simulink model "stability_controller_testbench"  (R2022b)
settings: Solver=VariableStepAuto  StartTime=0.0  StopTime=sim_t_stop  RelTol=1e-3
undefined symbols (not defined in the file): A, B, beta_off_deg, beta_on_deg, C, D, delta_base_deg, delta_base_t_on, delta_extra_deg, delta_extra_t_off, delta_extra_t_on, G_rref, Ki_beta, Ki_r, Kp_beta, Kp_r, Mz_max, Mz_min, psi0, Vx_scenario, X0, x0_lat, Y0
libraries: slpidlib x2
settings Model: Creator=joseg  LastModifiedBy=joseg
settings OptimizationCC: ReuseModelBlockBuffer=on

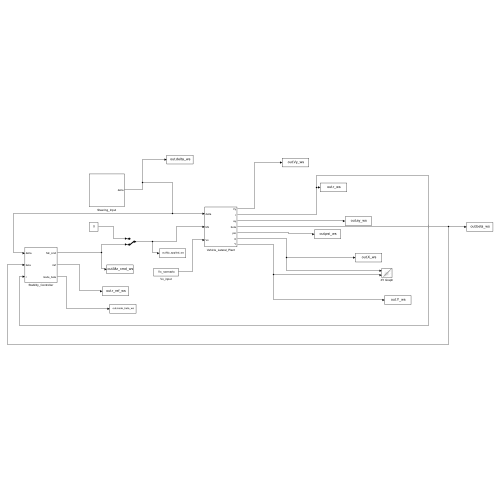
[thumbnail: Simulink's stored preview of the top-level diagram]
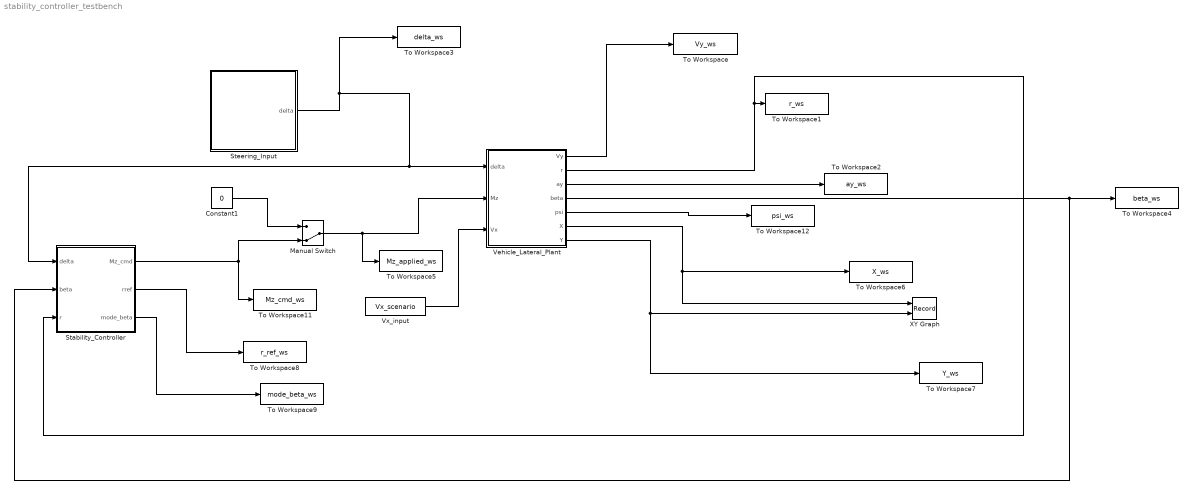
== system stability_controller_testbench ==
  Constant1 : Constant  Value=0
  Manual Switch : ManualSwitch  CurrentSetting=0
  Stability_Controller : Subsystem
  Steering_Input : Subsystem
  To Workspace : ToWorkspace  VariableName=Vy_ws  SaveFormat=Structure With Time  SampleTime=-1
      settings: Save2DSignal=2-D array (concatenate along first dimension)
  To Workspace1 : ToWorkspace  VariableName=r_ws  SaveFormat=Structure With Time  SampleTime=-1
      settings: Save2DSignal=2-D array (concatenate along first dimension)
  To Workspace11 : ToWorkspace  VariableName=Mz_cmd_ws  SaveFormat=Structure With Time  SampleTime=-1
      settings: Save2DSignal=2-D array (concatenate along first dimension)
  To Workspace12 : ToWorkspace  VariableName=psi_ws  SaveFormat=Structure With Time  SampleTime=-1
      settings: Save2DSignal=2-D array (concatenate along first dimension)
  To Workspace2 : ToWorkspace  VariableName=ay_ws  SaveFormat=Structure With Time  SampleTime=-1
      settings: Save2DSignal=2-D array (concatenate along first dimension)
  To Workspace3 : ToWorkspace  VariableName=delta_ws  SaveFormat=Structure With Time  SampleTime=-1
      settings: Save2DSignal=2-D array (concatenate along first dimension)
  To Workspace4 : ToWorkspace  VariableName=beta_ws  SaveFormat=Structure With Time  SampleTime=-1
      settings: Save2DSignal=2-D array (concatenate along first dimension)
  To Workspace5 : ToWorkspace  VariableName=Mz_applied_ws  SaveFormat=Structure With Time  SampleTime=-1
      settings: Save2DSignal=2-D array (concatenate along first dimension)
  To Workspace6 : ToWorkspace  VariableName=X_ws  SaveFormat=Structure With Time  SampleTime=-1
      settings: Save2DSignal=2-D array (concatenate along first dimension)
  To Workspace7 : ToWorkspace  VariableName=Y_ws  SaveFormat=Structure With Time  SampleTime=-1
      settings: Save2DSignal=2-D array (concatenate along first dimension)
  To Workspace8 : ToWorkspace  VariableName=r_ref_ws  SaveFormat=Structure With Time  SampleTime=-1
      settings: Save2DSignal=2-D array (concatenate along first dimension)
  To Workspace9 : ToWorkspace  VariableName=mode_beta_ws  SaveFormat=Structure With Time  SampleTime=-1
      settings: Save2DSignal=2-D array (concatenate along first dimension)
  Vehicle_Lateral_Plant : Subsystem
  Vx_input : Constant  Value=Vx_scenario
  XY Graph : Record  FileSettingsInternal="{\"entries\":[{\"content\":{\"excelSettings\":{\"content\":{},\"type\":\"Streamout.ExcelSettings\"}},\"type\":\"Streamout.FileSettingStorage\",\"uuid\":\"\"}],\"packageUris\":[\"http:\\/\\/schema.mathworks.com\\/mf0\\/streamout_blocks\\/R2020a\"],\"version\":\"1.0\"}"  Layout=[1 1]  SignalsInternal="{\"entries\":[{\"content\":{\"signals\":[{\"content\":{\"blockPath\":[],\"dimensions\":[1],\"domain\":\"\",\"lineColor\":\"#77ac30\",\"port\":1,\"signalID\":1,\"signalName\":\"Vehicle_Lateral_Plant:6\"},\"type\":\"RecordBlkView.Signal\",\"uuid\":\"\"},{\"content\":{\"blockPath\":[],\"dimensions\":[1],\"domain\":\"\",\"lineColor\":\"#4dbeee\",\"port\":2,\"signalID\":2,\"signalName\":\"Vehicle_Lateral_Plant:7\"},\"type\":\"RecordBlkView.Signal\",\"uuid\":\"\"}]},\"type\":\"RecordBlkView.InputSignals\",\"uuid\":\"\"}],\"packageUris\":[\"http:\\/\\/schema.mathworks.com\\/mf0\\/streamout_blocks\\/R2020a\"],\"version\":\"1.0\"}"  VisualizationBindings="{\"xyplotplugin\":{\"info\":[{\"series\":[],\"subplotID\":1}]}}"  CompatibilityTag=XY
  wires:
  Steering_Input/1(delta) -> To Workspace3/1, Stability_Controller/1(delta), Vehicle_Lateral_Plant/1(delta)
  Vehicle_Lateral_Plant/4(beta) -> Stability_Controller/2(beta), To Workspace4/1
  Vehicle_Lateral_Plant/7(Y) -> XY Graph/2, To Workspace7/1
  Vehicle_Lateral_Plant/1(Vy) -> To Workspace/1
  Vehicle_Lateral_Plant/6(X) -> XY Graph/1, To Workspace6/1
  Vehicle_Lateral_Plant/3(ay) -> To Workspace2/1
  Vx_input/1 -> Vehicle_Lateral_Plant/3(Vx)
  Vehicle_Lateral_Plant/5(psi) -> To Workspace12/1
  Stability_Controller/1(Mz_cmd) -> Manual Switch/2, To Workspace11/1
  Stability_Controller/2(rref) -> To Workspace8/1
  Stability_Controller/3(mode_beta) -> To Workspace9/1
  Vehicle_Lateral_Plant/2(r) -> Stability_Controller/3(r), To Workspace1/1
  Constant1/1 -> Manual Switch/1
  Manual Switch/1 -> To Workspace5/1, Vehicle_Lateral_Plant/2(Mz)

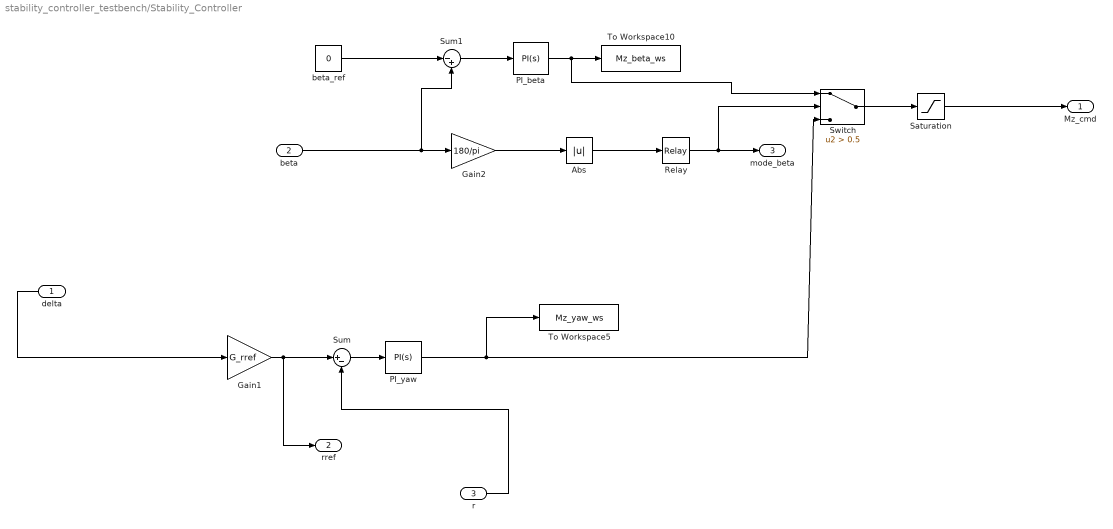
== system stability_controller_testbench/Stability_Controller ==
  delta : Inport
  beta : Inport  Port=2
  r : Inport  Port=3
  Abs : Abs  SaturateOnIntegerOverflow=off
  Gain1 : Gain  Gain=G_rref
  Gain2 : Gain  Gain=180/pi
  PI_beta : slpidlib/PID Controller  Controller=PI  Form=Parallel  TimeDomain=Continuous-time  UseExternalTs=off  SampleTime=-1  IntegratorMethod=Forward Euler  FilterMethod=Forward Euler  ControllerParametersSource=internal  P=Kp_beta  I=Ki_beta  UseKiTs=off  D=0  N=100  UseFilter=on  TunerSelectOption=Transfer Function Based (PID Tuner App)  InitialConditionSource=internal  InitialConditionForIntegrator=0  InitialConditionForFilter=0  DifferentiatorICPrevScaledInput=0  ExternalReset=none  TrackingMode=off  Kt=1  LimitOutput=off  SatLimitsSource=internal  UpperSaturationLimit=inf  LowerSaturationLimit=-inf  LinearizeAsGain=on  AntiWindupMode=none  Kb=1  LimitIntegrator=off  UpperIntegratorSaturationLimit=inf  LowerIntegratorSaturationLimit=-inf  POutMin=[]  POutMax=[]  IOutMin=[]  IOutMax=[]  DOutMin=[]  DOutMax=[]  NOutMin=[]  NOutMax=[]  SumOutMin=[]  SumOutMax=[]  SaturationOutMin=[]  SaturationOutMax=[]  PParamMin=[]  PParamMax=[]  IParamMin=[]  IParamMax=[]  DParamMin=[]  DParamMax=[]  NParamMin=[]  NParamMax=[]  KbParamMin=[]  KbParamMax=[]  KtParamMin=[]  KtParamMax=[]  KbOutMin=[]  KbOutMax=[]  KtOutMin=[]  KtOutMax=[]  IntegratorOutMin=[]  IntegratorOutMax=[]  FilterOutMin=[]  FilterOutMax=[]  SumI1OutMin=[]  SumI1OutMax=[]  SumI2OutMin=[]  SumI2OutMax=[]  SumI3OutMin=[]  SumI3OutMax=[]  SumI4OutMin=[]  SumI4OutMax=[]  SumDOutMin=[]  SumDOutMax=[]  DifferentiatorOutMin=[]  DifferentiatorOutMax=[]  FilterDiffOutCoefMin=[]  FilterDiffOutCoefMax=[]  ReciprocalOutMin=[]  ReciprocalOutMax=[]  SumDenOutMin=[]  SumDenOutMax=[]  SumNumOutMin=[]  SumNumOutMax=[]  DivideOutMin=[]  DivideOutMax=[]  UdiffTsProdOutMin=[]  UdiffTsProdOutMax=[]  NTsProdOutMin=[]  NTsProdOutMax=[]  UintegralTsProdOutMin=[]  UintegralTsProdOutMax=[]  UngainTsProdOutMin=[]  UngainTsProdOutMax=[]  IntegratorContinuousStateAttributes=''  IntegratorStateMustResolveToSignalObject=off  IntegratorRTWStateStorageClass=Auto  FilterContinuousStateAttributes=''  FilterStateMustResolveToSignalObject=off  FilterRTWStateStorageClass=Auto  ParallelPVariant=InternalParameters  IdealPVariant=Disabled  IVariant=InternalParameters  DVariant=Disabled  IntegratorVariant=Continuous  SatVariant=Disabled  AWVariant=Passthrough  PCopyVariant=Disabled  TRVariant=Disabled  FdbkBlocksVariant=Forward  IdealPFdbkVariant=Disabled  SatFdbkVariant=Disabled  DerivativeFilterVariant=Disabled  NVariant=Disabled  NCopyVariant=Disabled_SignalSpec  FilterICVariant=Disabled  IntegratorICVariant=InternalICs  ExternalResetVariant=Disabled  TRSumVariant=Passthrough  SumFdbkVariant=Disabled  SumVariant=Sum_PI  TsampFilterVariant=InternalTs  TsampNgainVariant=Passthrough  TsampIntegralVariant=Disabled_SignalSpec  ExternalSaturationOutDataTypeStr=Inherit: Same as second input
  PI_yaw : slpidlib/PID Controller  Controller=PI  Form=Parallel  TimeDomain=Continuous-time  UseExternalTs=off  SampleTime=-1  IntegratorMethod=Forward Euler  FilterMethod=Forward Euler  ControllerParametersSource=internal  P=Kp_r  I=Ki_r  UseKiTs=off  D=0  N=100  UseFilter=on  TunerSelectOption=Transfer Function Based (PID Tuner App)  InitialConditionSource=internal  InitialConditionForIntegrator=0  InitialConditionForFilter=0  DifferentiatorICPrevScaledInput=0  ExternalReset=none  TrackingMode=off  Kt=1  LimitOutput=off  SatLimitsSource=internal  UpperSaturationLimit=inf  LowerSaturationLimit=-inf  LinearizeAsGain=on  AntiWindupMode=none  Kb=1  LimitIntegrator=off  UpperIntegratorSaturationLimit=inf  LowerIntegratorSaturationLimit=-inf  POutMin=[]  POutMax=[]  IOutMin=[]  IOutMax=[]  DOutMin=[]  DOutMax=[]  NOutMin=[]  NOutMax=[]  SumOutMin=[]  SumOutMax=[]  SaturationOutMin=[]  SaturationOutMax=[]  PParamMin=[]  PParamMax=[]  IParamMin=[]  IParamMax=[]  DParamMin=[]  DParamMax=[]  NParamMin=[]  NParamMax=[]  KbParamMin=[]  KbParamMax=[]  KtParamMin=[]  KtParamMax=[]  KbOutMin=[]  KbOutMax=[]  KtOutMin=[]  KtOutMax=[]  IntegratorOutMin=[]  IntegratorOutMax=[]  FilterOutMin=[]  FilterOutMax=[]  SumI1OutMin=[]  SumI1OutMax=[]  SumI2OutMin=[]  SumI2OutMax=[]  SumI3OutMin=[]  SumI3OutMax=[]  SumI4OutMin=[]  SumI4OutMax=[]  SumDOutMin=[]  SumDOutMax=[]  DifferentiatorOutMin=[]  DifferentiatorOutMax=[]  FilterDiffOutCoefMin=[]  FilterDiffOutCoefMax=[]  ReciprocalOutMin=[]  ReciprocalOutMax=[]  SumDenOutMin=[]  SumDenOutMax=[]  SumNumOutMin=[]  SumNumOutMax=[]  DivideOutMin=[]  DivideOutMax=[]  UdiffTsProdOutMin=[]  UdiffTsProdOutMax=[]  NTsProdOutMin=[]  NTsProdOutMax=[]  UintegralTsProdOutMin=[]  UintegralTsProdOutMax=[]  UngainTsProdOutMin=[]  UngainTsProdOutMax=[]  IntegratorContinuousStateAttributes=''  IntegratorStateMustResolveToSignalObject=off  IntegratorRTWStateStorageClass=Auto  FilterContinuousStateAttributes=''  FilterStateMustResolveToSignalObject=off  FilterRTWStateStorageClass=Auto  ParallelPVariant=InternalParameters  IdealPVariant=Disabled  IVariant=InternalParameters  DVariant=Disabled  IntegratorVariant=Continuous  SatVariant=Disabled  AWVariant=Passthrough  PCopyVariant=Disabled  TRVariant=Disabled  FdbkBlocksVariant=Forward  IdealPFdbkVariant=Disabled  SatFdbkVariant=Disabled  DerivativeFilterVariant=Disabled  NVariant=Disabled  NCopyVariant=Disabled_SignalSpec  FilterICVariant=Disabled  IntegratorICVariant=InternalICs  ExternalResetVariant=Disabled  TRSumVariant=Passthrough  SumFdbkVariant=Disabled  SumVariant=Sum_PI  TsampFilterVariant=InternalTs  TsampNgainVariant=Passthrough  TsampIntegralVariant=Disabled_SignalSpec  ExternalSaturationOutDataTypeStr=Inherit: Same as second input
  Relay : Relay  OnSwitchValue=beta_on_deg  OffSwitchValue=beta_off_deg
  Saturation : Saturate  UpperLimit=Mz_max  LowerLimit=Mz_min
  Sum : Sum  Inputs=|+-
  Sum1 : Sum  Inputs=|-+
  Switch : Switch  Criteria=u2 > Threshold  Threshold=0.5  SaturateOnIntegerOverflow=off  InputSameDT=off
  To Workspace10 : ToWorkspace  VariableName=Mz_beta_ws  SaveFormat=Structure With Time  SampleTime=-1
      settings: Save2DSignal=2-D array (concatenate along first dimension)
  To Workspace5 : ToWorkspace  VariableName=Mz_yaw_ws  SaveFormat=Structure With Time  SampleTime=-1
      settings: Save2DSignal=2-D array (concatenate along first dimension)
  beta_ref : Constant  Value=0
  Mz_cmd : Outport
  rref : Outport  Port=2
  mode_beta : Outport  Port=3
  wires:
  beta_ref/1 -> Sum1/1
  Abs/1 -> Relay/1
  PI_beta/1 -> Switch/1, To Workspace10/1
  beta/1 -> Sum1/2, Gain2/1
  PI_yaw/1 -> To Workspace5/1, Switch/3
  Gain2/1 -> Abs/1
  Sum/1 -> PI_yaw/1
  Sum1/1 -> PI_beta/1
  Gain1/1 -> rref/1, Sum/1
  delta/1 -> Gain1/1
  r/1 -> Sum/2
  Switch/1 -> Saturation/1
  Saturation/1 -> Mz_cmd/1
  Relay/1 -> Switch/2, mode_beta/1

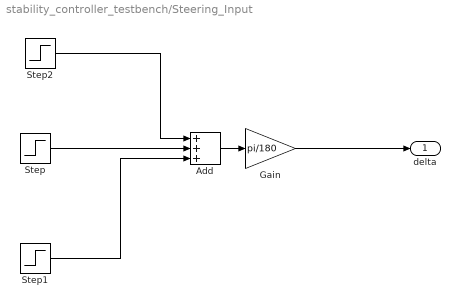
== system stability_controller_testbench/Steering_Input ==
  Add : Sum  Inputs=+++
  Gain : Gain  Gain=pi/180
  Step : Step  Time=delta_extra_t_on  After=delta_extra_deg  SampleTime=0
  Step1 : Step  Time=delta_extra_t_off  After=-delta_extra_deg  SampleTime=0
  Step2 : Step  Time=delta_base_t_on  After=delta_base_deg  SampleTime=0
  delta : Outport
  wires:
  Gain/1 -> delta/1
  Add/1 -> Gain/1
  Step2/1 -> Add/1
  Step/1 -> Add/2
  Step1/1 -> Add/3

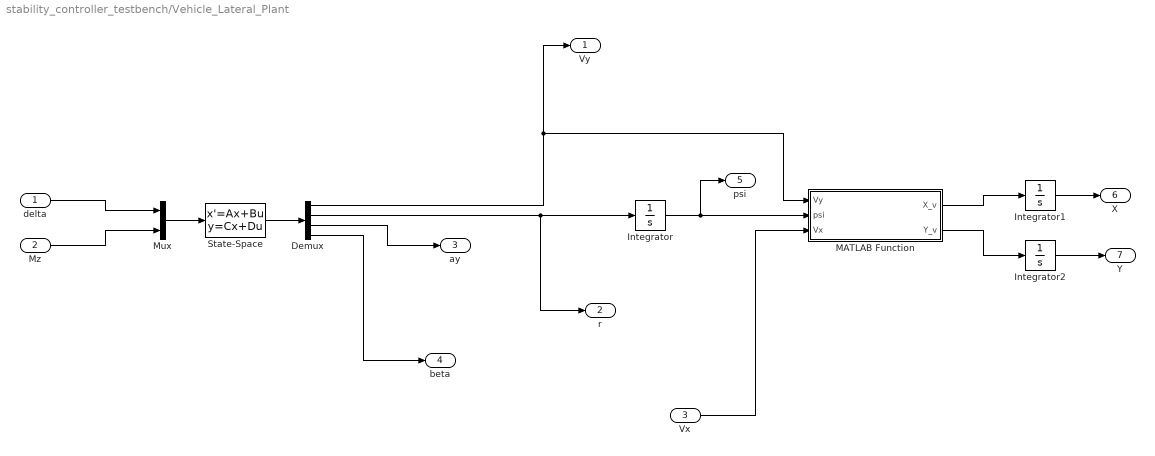
== system stability_controller_testbench/Vehicle_Lateral_Plant ==
  delta : Inport
  Mz : Inport  Port=2
  Vx : Inport  Port=3
  Demux : Demux
  Integrator : Integrator  InitialCondition=psi0
  Integrator1 : Integrator  InitialCondition=X0
  Integrator2 : Integrator  InitialCondition=Y0
  MATLAB Function : MATLAB Function  TreatAsAtomicUnit=on
  Mux : Mux  Inputs=2
  State-Space : StateSpace  A=A  B=B  C=C  D=D  InitialCondition=x0_lat
  Vy : Outport
  r : Outport  Port=2
  ay : Outport  Port=3
  beta : Outport  Port=4
  psi : Outport  Port=5
  X : Outport  Port=6
  Y : Outport  Port=7
  wires:
  Integrator/1 -> psi/1, MATLAB Function/2(psi)
  MATLAB Function/2(Y_v) -> Integrator2/1
  Demux/2 -> r/1, Integrator/1
  State-Space/1 -> Demux/1
  Vx/1 -> MATLAB Function/3(Vx)
  Demux/1 -> Vy/1, MATLAB Function/1(Vy)
  MATLAB Function/1(X_v) -> Integrator1/1
  Integrator2/1 -> Y/1
  Mux/1 -> State-Space/1
  Integrator1/1 -> X/1
  Demux/4 -> beta/1
  Demux/3 -> ay/1
  delta/1 -> Mux/1
  Mz/1 -> Mux/2

== matlab function stability_controller_testbench/Vehicle_Lateral_Plant/MATLAB Function ==
  data: Vy input; X_v output; psi input; Vx input; Y_v output
function [X_v, Y_v] = body_to_inertial(Vy, psi, Vx)
X_v = Vx*cos(psi) - Vy*sin(psi);
Y_v = Vx*sin(psi) + Vy*cos(psi);
end
